simulink model "VD_mpc"  (R2023a)
settings: Solver=VariableStepAuto  StartTime=0.0  StopTime=20  RelTol=1e-3
values from neighbouring files (symbols this model uses):
  Ts = 0.1    [MPC_main.m]    (also in mpc_closed_loop.m = 1)
libraries: mpclib x1
settings Model: Creator=swati  LastModifiedBy=swati
settings DebuggingCC: TimeAdjustmentMsg=warning  InheritedTsInSrcMsg=error

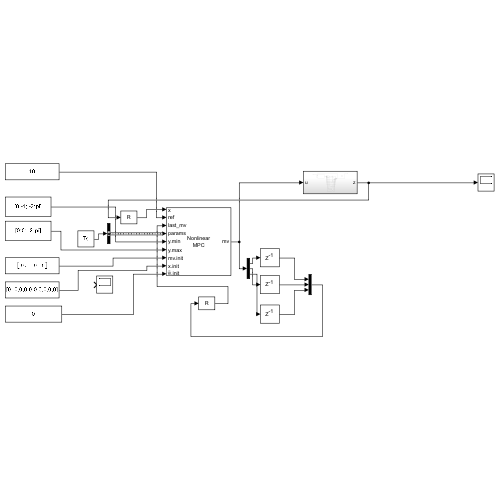
[thumbnail: Simulink's stored preview of the top-level diagram]
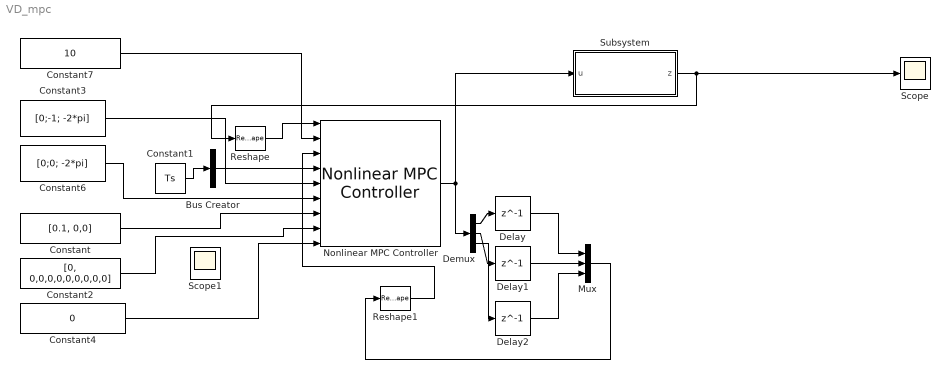
== system VD_mpc ==
  Bus Creator : BusCreator  Inputs=1  OutDataTypeStr=Bus: myBusObject  NonVirtualBus=on
      settings: InheritFromInputs=off
  Constant : Constant  Value=[0.1, 0,0]  VectorParams1D=off
  Constant1 : Constant  Value=Ts
  Constant2 : Constant  Value=[0, 0,0,0,0,0,0,0,0,0]  VectorParams1D=off
  Constant3 : Constant  Value=[0;-1; -2*pi]  VectorParams1D=off
  Constant4 : Constant  Value=0
  Constant6 : Constant  Value=[0;0; -2*pi]  VectorParams1D=off
  Constant7 : Constant  Value=10  VectorParams1D=off
  Delay : Delay  DelayLength=1  InitialCondition=0
  Delay1 : Delay  DelayLength=1  InitialCondition=0
  Delay2 : Delay  DelayLength=1  InitialCondition=0
  Demux : Demux  Outputs=3
  Mux : Mux  Inputs=3
  Nonlinear MPC Controller : mpclib/Nonlinear MPC Controller  nlmpcobj=nlobj  UseObjectTs=on  UseMEX=off  md_enabled=off  mvtarget_enabled=off  param_enabled=on  cost_enabled=off  mvseq_enabled=off  stateseq_enabled=off  ovseq_enabled=off  slack_enabled=off  status_enabled=off  ov_min=on  ov_max=on  mv_min=off  mv_max=off  mvrate_min=off  mvrate_max=off  state_min=off  state_max=off  ov_weight=off  mv_weight=off  mvrate_weight=off  ecr_weight=off  nlp_initialize=on
  Reshape : Reshape  OutputDimensionality=Customize  OutputDimensions=[1,10]
  Reshape1 : Reshape  OutputDimensionality=Customize  OutputDimensions=[1,3]
  Scope : Scope
  Scope1 : Scope
  Subsystem : Subsystem
  wires:
  Constant7/1 -> Nonlinear MPC Controller/2
  Subsystem/1(z) -> Reshape/1, Scope/1
  Nonlinear MPC Controller/1 -> Subsystem/1(u), Demux/1
  Constant1/1 -> Bus Creator/1
  Bus Creator/1 -> Nonlinear MPC Controller/4
  Demux/1 -> Delay/1
  Demux/2 -> Delay1/1
  Demux/3 -> Delay2/1
  Delay/1 -> Mux/1
  Delay1/1 -> Mux/2
  Delay2/1 -> Mux/3
  Mux/1 -> Reshape1/1
  Constant/1 -> Nonlinear MPC Controller/7
  Constant4/1 -> Nonlinear MPC Controller/9
  Constant2/1 -> Nonlinear MPC Controller/8
  Reshape/1 -> Nonlinear MPC Controller/1
  Constant3/1 -> Nonlinear MPC Controller/5
  Constant6/1 -> Nonlinear MPC Controller/6
  Reshape1/1 -> Nonlinear MPC Controller/3

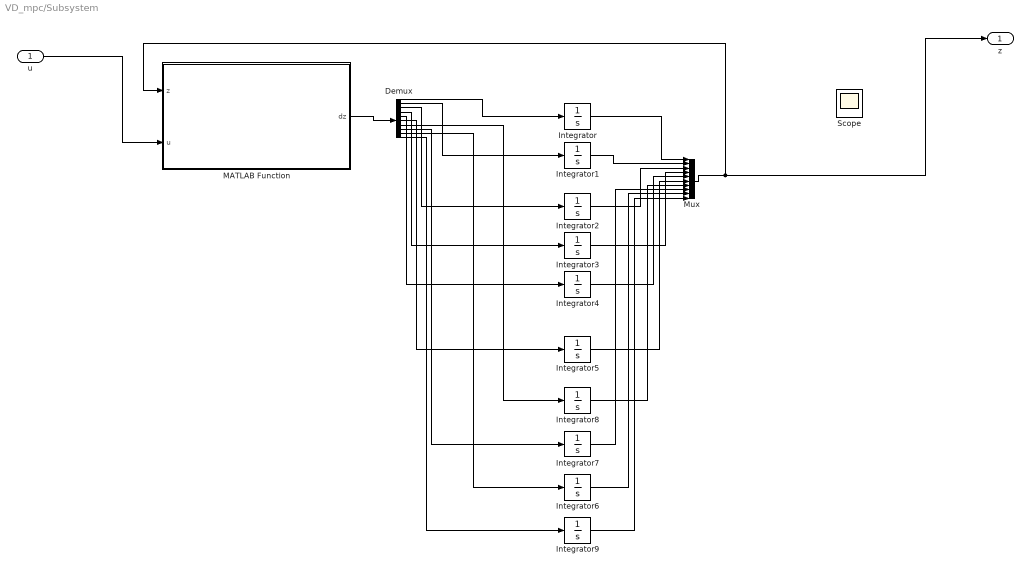
== system VD_mpc/Subsystem ==
  u : Inport
  Demux : Demux  Outputs=10
  Integrator{,1..9} (10 alike) : Integrator
  MATLAB Function : MATLAB Function  TreatAsAtomicUnit=on
  Mux : Mux  Inputs=10
  Scope : Scope
  z : Outport
  wires:
  u/1 -> MATLAB Function/2(u)
  MATLAB Function/1(dz) -> Demux/1
  Integrator/1 -> Mux/1
  Demux/1 -> Integrator/1
  Demux/2 -> Integrator1/1
  Demux/3 -> Integrator2/1
  Demux/4 -> Integrator3/1
  Demux/5 -> Integrator4/1
  Demux/6 -> Integrator5/1
  Demux/7 -> Integrator8/1
  Demux/8 -> Integrator7/1
  Demux/9 -> Integrator6/1
  Demux/10 -> Integrator9/1
  Integrator1/1 -> Mux/2
  Integrator2/1 -> Mux/3
  Integrator3/1 -> Mux/4
  Integrator4/1 -> Mux/5
  Integrator5/1 -> Mux/6
  Integrator8/1 -> Mux/7
  Integrator7/1 -> Mux/8
  Integrator6/1 -> Mux/9
  Integrator9/1 -> Mux/10
  Mux/1 -> MATLAB Function/1(z), z/1

== matlab function VD_mpc/Subsystem/MATLAB Function ==
  data: z input; u input; dz output
%Author: Swati V. Shirke
%This code is for state space of vehicle dynamics
% states: Vx, Vy, r

function dz = vehicle_dynamics( z, u)
    % abc = Forces
    % dt;
    %tic;
    dz= zeros(10,1);
    accel = u(1);
    deccel = u(2);
    delta = u(3); %(pi/180) * sin(2*pi*0.1*t); %
    params = system_parameters();
    Vx = z(1);
    Vy = z(2);
    r  = z(3);
    x  = z(4);
    y  = z(5);
    psi= z(6);
    ax = z(1) * r;
    ay = z(2) * r;

    %%input torue to each wheel 
    tau_in = cal_wheel_torque_in(params, accel, deccel);
    tau_in_fl = tau_in(1);
    tau_in_fr = tau_in(2);
    tau_in_rl = tau_in(3);
    tau_in_rr = tau_in(4);
    
    %% calculate forces
    t_forces = tire_forces(params, z, delta, ax, ay); %8 * 1 vector
    [Fx_sum, Fy_f, Fy_r, Fy_del] = vehicle_forces(params, z, t_forces, delta);
        
    Vx_dt = Vy * r + (Fx_sum / params.m);
    Vy_dt = -Vx * r + ((Fy_f+ Fy_r) / params.m);

    t_forces = tire_forces(params, z, delta, Vx_dt, Vy_dt); %8 * 1 vector
    [Fx_sum, Fy_f, Fy_r, Fy_del] = vehicle_forces(params, z, t_forces, delta);


    Vx_dt = Vy * r + (Fx_sum / params.m);
    Vy_dt = -Vx * r + ((Fy_f+ Fy_r) / params.m);
    r_dt =  (params.a * Fy_f - params.b *Fy_r + Fy_del) / params.Izz_v;

    x_dt = Vx * cos(psi) - Vy * sin(psi);
    y_dt = Vx * sin(psi) + Vy * cos(psi);
    psi_dt  = r;
    
    

    %set tire forces 
    Fx_fl = t_forces(1);
    Fx_fr = t_forces(2);
    Fx_rl = t_forces(3);
    Fx_rr = t_forces(4); 

    %wheel velocities 
    w_fl_dt = (tau_in_fl - Fx_fl * params.R_f) / params.Iyy_w_f;
    w_fr_dt = (tau_in_fr - Fx_fr * params.R_f) / params.Iyy_w_f;
    w_rl_dt = (tau_in_rl - Fx_rl * params.R_r) / params.Iyy_w_r;
    w_rr_dt = (tau_in_rr - Fx_rr * params.R_r) / params.Iyy_w_r;

    omega_fl_dt = w_fl_dt;
    omega_fr_dt = w_fr_dt;
    omega_rl_dt = w_rl_dt;
    omega_rr_dt = w_rr_dt;
    %tp = toc;
    dz = [Vx_dt; Vy_dt; r_dt; x_dt; y_dt; psi_dt; omega_fl_dt; omega_fr_dt; omega_rl_dt; omega_rr_dt];

    % ax = (Vx_dt -ax)/dt;
    % ay = (Vy_dt - ay)/dt;
    % 
    %dz = [Vx_dt; Vy_dt; r_dt; x_dt; y_dt; psi_dt; omega_fl_dt; omega_fr_dt; omega_rl_dt; omega_rr_dt; ax; ay];


end
